simulink model "vco_counter"  (R2019b)
settings: Solver=VariableStepAuto  StartTime=0.0  StopTime=1e-8  RelTol=1e-3
values from neighbouring files (symbols this model uses):
  fs = fB*2    (= 10000000)    [vco_counter_m.m]    (also in vco_m.m = 1600000000)
  fsig = 1.3e6    (= 1300000)    [vco_counter_m.m]    (also in vco_m.m = 13000000)
  ts = 1/fs    (= 1e-07)    [vco_counter_m.m]    (also in vco_m.m = 6.25e-10)
  tsys_res = 1e-11    [vco_counter_m.m]    (also in vco_m.m = 6.25e-10)
libraries: commsynccomp2 x1, dspswit3 x1, dspbuff3 x1, dspsigops x1
settings Model: Creator=benve  LastModifiedBy=benve

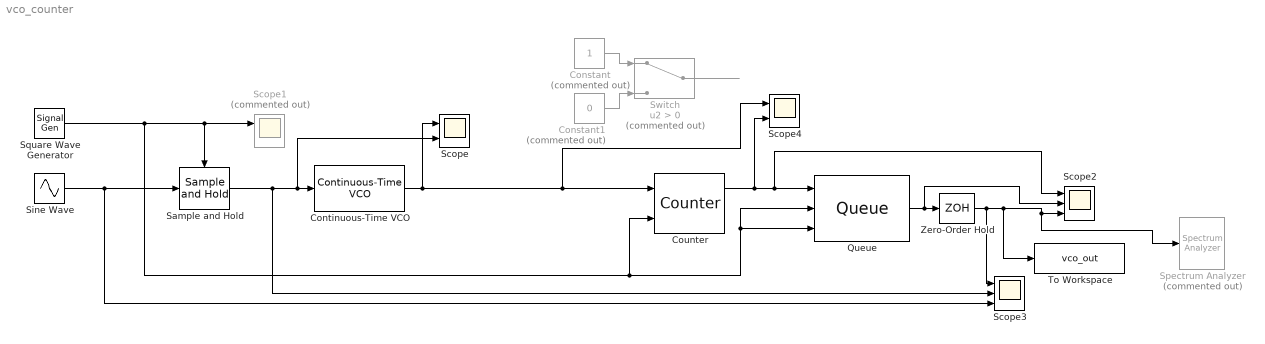
== system vco_counter ==
  Constant : Constant  Commented=on
  Constant1 : Constant  Commented=on  Value=0
  Continuous-Time VCO : commsynccomp2/Continuous-Time VCO  Ac=1  Fc=fvco  Kc=fsens  Ph=0
      settings: SourceProductName=Communications Toolbox  SourceProductBaseCode=CM
  Counter : dspswit3/Counter  Direction=Up  CountEvent=Rising edge  CounterSize=User defined  MaxCount=65535  InitialCount=0  Output=Count and Hit  HitValue=32  ResetInput=on  SamplesPerFrame=1  Ts=1  CntDtype=double  HitDtype=Logical
  Queue : dspbuff3/Queue  depth=8  trigger=Rising edge  overflow=Dynamic reallocation  pes=Warning  eso=off  fso=off  nso=off  clr=off  clrOutport=off  adf=on
      settings: SourceProductName=DSP System Toolbox  SourceProductBaseCode=DS
  Sample and Hold : dspsigops/Sample and Hold  trig=Rising edge  initCond=0  latchinput=off
  Scope : Scope  NumInputPorts=2
  Scope1 : Scope  Commented=on  NumInputPorts=2
  Scope2 : Scope  NumInputPorts=3
  Scope3 : Scope  NumInputPorts=3
  Scope4 : Scope  NumInputPorts=2
  Sine Wave : Sin  Frequency=fsig*2*pi  SampleTime=tsys_res
  Spectrum Analyzer : SpectrumAnalyzer  Commented=on
  Square Wave Generator : SignalGenerator  WaveForm=square  Frequency=fs
  Switch : Switch  Commented=on  Criteria=u2 > Threshold
  To Workspace : ToWorkspace  VariableName=vco_out  SampleTime=-1
      settings: Save2DSignal=2-D array (concatenate along first dimension)
  Zero-Order Hold : ZeroOrderHold  SampleTime=ts
  wires:
  Sample and Hold/1 -> Scope3/2, Scope/2, Continuous-Time VCO/1
  Continuous-Time VCO/1 -> Scope4/1, Counter/1, Scope/1
  Counter/1 -> Scope4/2, Scope2/1, Queue/1
  Square Wave Generator/1 -> Queue/2, Queue/3, Counter/2, Scope1/1, Sample and Hold/Trigger
  Zero-Order Hold/1 -> Scope3/1, To Workspace/1, Spectrum Analyzer/1, Scope2/3
  Sine Wave/1 -> Sample and Hold/1, Scope3/3
  Queue/1 -> Zero-Order Hold/1, Scope2/2
  Constant/1 -> Switch/1
  ? -> Switch/2
  Constant1/1 -> Switch/3
  Switch/1 -> ?
